simulink model "dead_zone"  (R2021a)
settings: Solver=VariableStepAuto  StartTime=0.0  StopTime=10.0  RelTol=1e-3
libraries: simulink x1
settings Model: Creator=DELL  LastModifiedBy=DELL

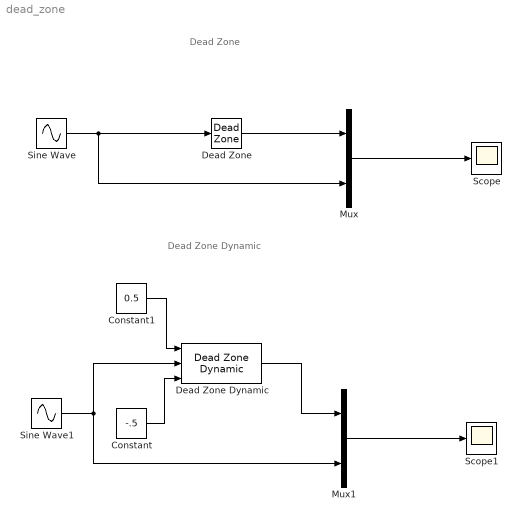
== system dead_zone ==
  note: Dead Zone
  note: Dead Zone Dynamic
  Constant : Constant  Value=-.5
  Constant1 : Constant  Value=0.5
  Dead Zone : DeadZone  SaturateOnIntegerOverflow=on
  Dead Zone Dynamic : simulink/Discontinuities/Dead Zone Dynamic
      settings: SourceProductBaseCode=SL
  Mux : Mux  Inputs=2
  Mux1 : Mux  Inputs=2
  Scope : Scope
  Scope1 : Scope
  Sine Wave : Sin  SampleTime=0
  Sine Wave1 : Sin  SampleTime=0
  wires:
  Sine Wave/1 -> Mux/2, Dead Zone/1
  Dead Zone/1 -> Mux/1
  Mux/1 -> Scope/1
  Mux1/1 -> Scope1/1
  Sine Wave1/1 -> Dead Zone Dynamic/2, Mux1/2
  Dead Zone Dynamic/1 -> Mux1/1
  Constant/1 -> Dead Zone Dynamic/3
  Constant1/1 -> Dead Zone Dynamic/1
